simulink model "model4"  (R2025a)
settings: Solver=VariableStepAuto  StartTime=0.0  StopTime=10  RelTol=1e-3
undefined symbols (not defined in the file): A, Aw, B, C, Cw, K, kr, Lw, Lx, R
settings Model: Creator=neso  LastModifiedBy=Nenad

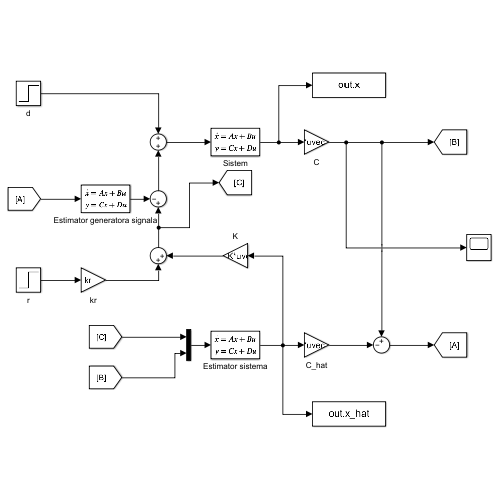
[thumbnail: Simulink's stored preview of the top-level diagram]
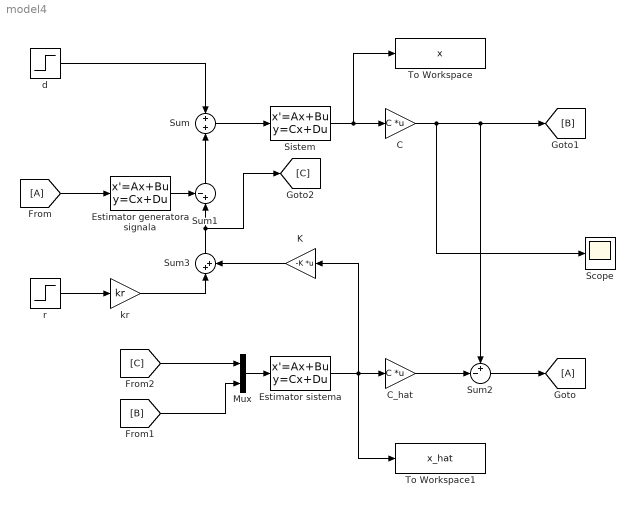
== system model4 ==
  C : Gain  Gain=C  Multiplication=Matrix(K*u) (u vector)
  C_hat : Gain  Gain=C  Multiplication=Matrix(K*u) (u vector)
  Estimator generatora signala : StateSpace  A=Aw  B=Lw  C=Cw  D=0  InitialCondition=0
  Estimator sistema : StateSpace  A=A - Lx * C  B=[B, Lx]  C=[1, 0; 0, 1]  D=[0, 0; 0, 0]  InitialCondition=0
  From : From
  Goto : Goto
  K : Gain  Gain=-K  Multiplication=Matrix(K*u) (u vector)
  Mux : Mux  Inputs=2
  Scope : Scope
      settings: ActiveDisplayYMinimum=-2.8746497894826097  ActiveDisplayYMaximum=5.8718481053434868
  Sistem : StateSpace  A=A  B=B  C=[1, 0; 0, 1]  D=[0; 0]  InitialCondition=[-2; -2]
  Sum : Sum  Inputs=+|+
  Sum1 : Sum  Inputs=-+|
  Sum2 : Sum  Inputs=+-|
  Sum3 : Sum  Inputs=|++
  To Workspace : ToWorkspace  VariableName=x  SaveFormat=Timeseries  SampleTime=-1
  To Workspace1 : ToWorkspace  VariableName=x_hat  SaveFormat=Timeseries  SampleTime=-1
  d : Step  Time=0  SampleTime=0
  kr : Gain  Gain=kr
  r : Step  Time=0  After=R  SampleTime=0
  wires:
  d/1 -> Sum/1
  Sum/1 -> Sistem/1
  Estimator sistema/1 -> To Workspace1/1, K/1, C_hat/1
  C_hat/1 -> Sum2/2
  Sum2/1 -> Goto/1
  From/1 -> Estimator generatora signala/1
  Mux/1 -> Estimator sistema/1
  [B] -> Mux/2
  [C] -> Mux/1
  Sistem/1 -> To Workspace/1, C/1
  C/1 -> Scope/1, Sum2/1, [B]
  r/1 -> kr/1
  Sum1/1 -> Sum/2
  Sum3/1 -> [C], Sum1/2
  K/1 -> Sum3/2
  kr/1 -> Sum3/1
  Estimator generatora signala/1 -> Sum1/1
